simulink model "hybrid_system"  (R2020b)
settings: Solver=FixedStepAuto  StartTime=0.0  StopTime=10.0  FixedStep=0.0001  RelTol=1e-3
settings Model: Creator=avina  LastModifiedBy=avina

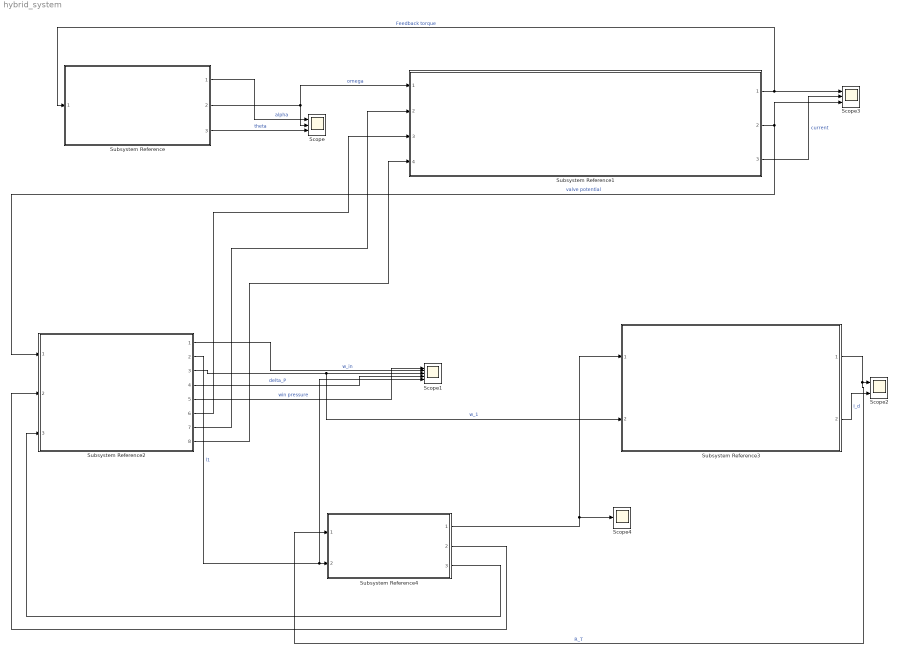
== system hybrid_system ==
  Scope : Scope  NumInputPorts=3
  Scope1 : Scope  NumInputPorts=5
  Scope2 : Scope  NumInputPorts=2
  Scope3 : Scope  NumInputPorts=3
  Scope4 : Scope
  Subsystem Reference : Subsystem  ReferencedSubsystem=Pendulum
  Subsystem Reference1 : Subsystem  ReferencedSubsystem=Motor_circuit
  Subsystem Reference2 : Subsystem  ReferencedSubsystem=Tank_system
  Subsystem Reference3 : Subsystem  ReferencedSubsystem=Dissipator_circuit
  Subsystem Reference4 : Subsystem  ReferencedSubsystem=coders4Avinash2
  wires:
  Subsystem Reference2/7 -> Subsystem Reference1/2
  Subsystem Reference2/6 -> Subsystem Reference1/3
  Subsystem Reference1/3 -> Scope3/2  "current"
  Subsystem Reference/3 -> Scope/3  "theta"
  Subsystem Reference2/8 -> Subsystem Reference1/4
  Subsystem Reference3/1 -> Subsystem Reference4/1, Scope2/1  "R_T"
  Subsystem Reference1/1 -> Subsystem Reference/1, Scope3/1  "Feedback torque"
  Subsystem Reference2/3 -> Subsystem Reference3/2, Scope1/3  "w_1"
  Subsystem Reference2/4 -> Scope1/4  "delta_P"
  Subsystem Reference/1 -> Scope/1  "alpha"
  Subsystem Reference/2 -> Scope/2, Subsystem Reference1/1  "omega"
  Subsystem Reference2/1 -> Scope1/2  "w_in"
  Subsystem Reference1/2 -> Scope3/3, Subsystem Reference2/1  "valve potential"
  Subsystem Reference4/3 -> Subsystem Reference2/3
  Subsystem Reference4/2 -> Subsystem Reference2/2
  Subsystem Reference2/5 -> Scope1/1  "win pressure"
  Subsystem Reference4/1 -> Subsystem Reference3/1, Scope4/1
  Subsystem Reference3/2 -> Scope2/2  "I_d"
  Subsystem Reference2/2 -> Scope1/5, Subsystem Reference4/2  "l1"
